simulink library "AVR_library"  (R2015b)
settings: Solver=VariableStepAuto  StartTime=0.0  StopTime=10.0  RelTol=1e-3
undefined symbols (not defined in the file): num_modes
settings Model: Creator=Paolo  LastModifiedBy=Paolo

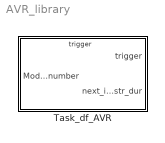
== system AVR_library ==
  Task_df_AVR : Subsystem  mask{conf_name=tAVR_instrs, num_modes=num_modes}
      mask prompts: conf_name "Task name"; num_modes "Number of modes"
      mask init:
      | set_param(sprintf('%s/task_AVR',gcb),'Parameters','conf_name num_modes')

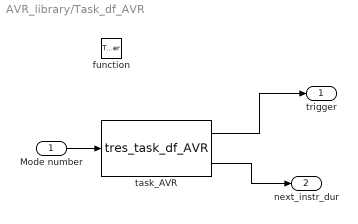
== system AVR_library/Task_df_AVR ==
  Mode number : Inport
  function : TriggerPort  TriggerType=function-call
  task_AVR : S-Function  FunctionName=tres_task_df_AVR  Parameters=conf_name num_modes  SFunctionDeploymentMode=off  EnableBusSupport=off
  trigger : Outport  OutputWhenDisabled=reset  InitialOutput=0.0
  next_instr_dur : Outport  Port=2
  wires:
  task_AVR/2 -> next_instr_dur/1
  task_AVR/1 -> trigger/1
  Mode number/1 -> task_AVR/1
